simulink model "bicycle_model"  (R2021a)
settings: Solver=FixedStepDiscrete  StartTime=0.0  StopTime=365  FixedStep=0.05  RelTol=1e-3
values from neighbouring files (symbols this model uses):
  L = 2.2    [changing_ld.m]    (also in params.m)
  Ld = 10    [changing_ld.m]    (also in params.m = 5)
  v = 1.0    (= 1)    [changing_ld.m]    (also in params.m)
  waypoints = [       0    0 ... (first row only)    [changing_ld.m]    (also in params.m)
undefined symbols (not defined in the file or in its folder): DiscIntNeverNeededParam
settings Model: Creator=Sıla The Magnificent  LastModifiedBy=Sıla The Magnificent

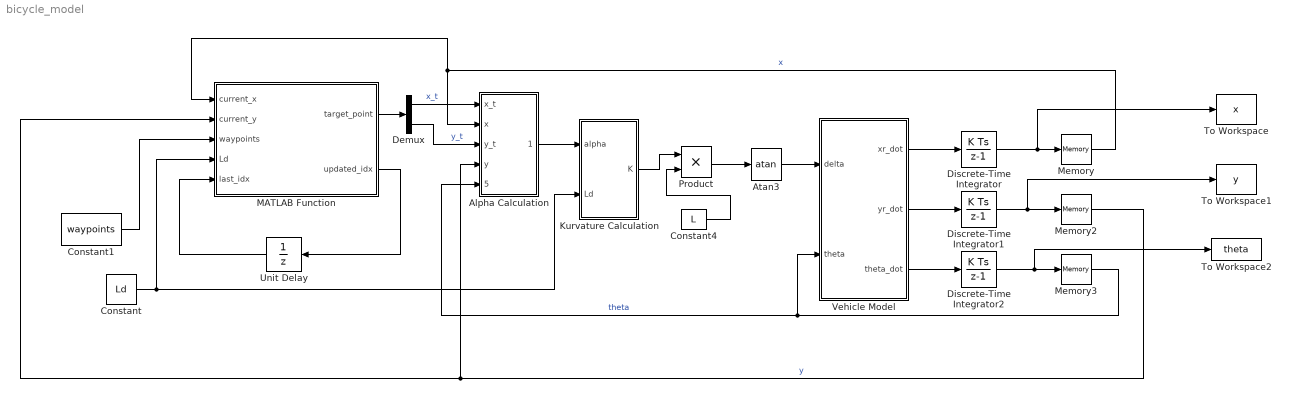
== system bicycle_model ==
  Alpha Calculation : Subsystem
  Atan3 : Trigonometry  Operator=atan
  Constant : Constant  Value=Ld
  Constant1 : Constant  Value=waypoints  SampleTime=0.05
  Constant4 : Constant  Value=L
  Demux : Demux  Outputs=2
  Discrete-Time Integrator : DiscreteIntegrator  SampleTime=0.05  ICPrevOutput=DiscIntNeverNeededParam  ICPrevScaledInput=DiscIntNeverNeededParam
  Discrete-Time Integrator1 : DiscreteIntegrator  SampleTime=0.05  ICPrevOutput=DiscIntNeverNeededParam  ICPrevScaledInput=DiscIntNeverNeededParam
  Discrete-Time Integrator2 : DiscreteIntegrator  SampleTime=0.05  ICPrevOutput=DiscIntNeverNeededParam  ICPrevScaledInput=DiscIntNeverNeededParam
  Kurvature Calculation : Subsystem
  MATLAB Function : MATLAB Function  TreatAsAtomicUnit=on  SystemSampleTime=0.05
  Memory : Memory  InheritSampleTime=on
  Memory2 : Memory  InheritSampleTime=on
  Memory3 : Memory  InheritSampleTime=on
  Product : Product
  To Workspace : ToWorkspace  VariableName=x  SaveFormat=Timeseries  SampleTime=-1
  To Workspace1 : ToWorkspace  VariableName=y  SaveFormat=Timeseries  SampleTime=-1
  To Workspace2 : ToWorkspace  VariableName=theta  SaveFormat=Timeseries  SampleTime=-1
  Unit Delay : UnitDelay  InitialCondition=2  SampleTime=0.05  HasFrameUpgradeWarning=on
  Vehicle Model : Subsystem
  wires:
  Vehicle Model/1(xr_dot) -> Discrete-Time Integrator/1
  Vehicle Model/2(yr_dot) -> Discrete-Time Integrator1/1
  Vehicle Model/3(theta_dot) -> Discrete-Time Integrator2/1
  Discrete-Time Integrator/1 -> To Workspace/1, Memory/1
  Memory/1 -> Alpha Calculation/2(x), MATLAB Function/1(current_x)  "x"
  Discrete-Time Integrator1/1 -> Memory2/1, To Workspace1/1
  Memory2/1 -> Alpha Calculation/4(y), MATLAB Function/2(current_y)  "y"
  Discrete-Time Integrator2/1 -> Memory3/1, To Workspace2/1
  Memory3/1 -> Vehicle Model/2(theta), Alpha Calculation/5(theta)  "theta"
  Product/1 -> Atan3/1
  Atan3/1 -> Vehicle Model/1(delta)
  Constant1/1 -> MATLAB Function/3(waypoints)
  Constant/1 -> MATLAB Function/4(Ld), Kurvature Calculation/2(Ld)
  MATLAB Function/2(updated_idx) -> Unit Delay/1
  Unit Delay/1 -> MATLAB Function/5(last_idx)
  MATLAB Function/1(target_point) -> Demux/1
  Demux/1 -> Alpha Calculation/1(x_t)  "x_t"
  Alpha Calculation/1(alpha) -> Kurvature Calculation/1(alpha)
  Demux/2 -> Alpha Calculation/3(y_t)  "y_t"
  Kurvature Calculation/1(K) -> Product/1
  Constant4/1 -> Product/2

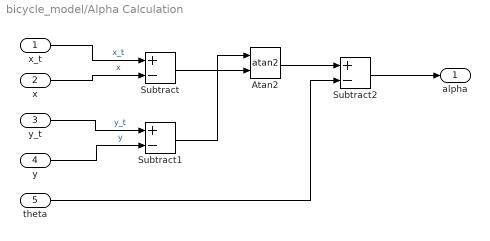
== system bicycle_model/Alpha Calculation ==
  x_t : Inport
  x : Inport  Port=2
  y_t : Inport  Port=3
  y : Inport  Port=4
  theta : Inport  Port=5
  Atan2 : Trigonometry  Operator=atan2
  Subtract : Sum  Inputs=+-
  Subtract1 : Sum  Inputs=+-
  Subtract2 : Sum  Inputs=+-
  alpha : Outport
  wires:
  x_t/1 -> Subtract/1  "x_t"
  Atan2/1 -> Subtract2/1
  x/1 -> Subtract/2  "x"
  y/1 -> Subtract1/2  "y"
  Subtract1/1 -> Atan2/1
  Subtract/1 -> Atan2/2
  Subtract2/1 -> alpha/1
  y_t/1 -> Subtract1/1  "y_t"
  theta/1 -> Subtract2/2

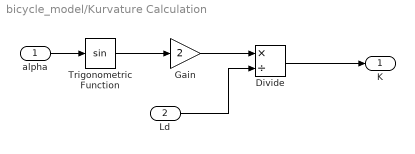
== system bicycle_model/Kurvature Calculation ==
  alpha : Inport
  Ld : Inport  Port=2
  Divide : Product  Inputs=*/
  Gain : Gain  Gain=2
  Trigonometric Function : Trigonometry
  K : Outport
  wires:
  Gain/1 -> Divide/1
  Ld/1 -> Divide/2
  Divide/1 -> K/1
  Trigonometric Function/1 -> Gain/1
  alpha/1 -> Trigonometric Function/1

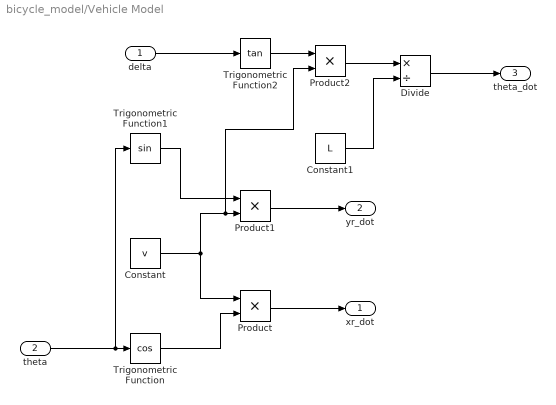
== system bicycle_model/Vehicle Model ==
  delta : Inport  OutMin=-0.5236  OutMax=0.5236
  theta : Inport  Port=2
  Constant : Constant  Value=v
  Constant1 : Constant  Value=L
  Divide : Product  Inputs=*/
  Product : Product
  Product1 : Product
  Product2 : Product
  Trigonometric Function : Trigonometry  Operator=cos
  Trigonometric Function1 : Trigonometry
  Trigonometric Function2 : Trigonometry  Operator=tan
  xr_dot : Outport
  yr_dot : Outport  Port=2
  theta_dot : Outport  Port=3
  wires:
  Trigonometric Function1/1 -> Product1/1
  Constant/1 -> Product2/2, Product1/2, Product/1
  Trigonometric Function/1 -> Product/2
  theta/1 -> Trigonometric Function1/1, Trigonometric Function/1
  delta/1 -> Trigonometric Function2/1
  Product/1 -> xr_dot/1
  Trigonometric Function2/1 -> Product2/1
  Product1/1 -> yr_dot/1
  Product2/1 -> Divide/1
  Constant1/1 -> Divide/2
  Divide/1 -> theta_dot/1

== matlab function bicycle_model/MATLAB Function ==
  data: current_x input; target_point output; current_y input; waypoints input; Ld input; updated_idx output; last_idx input
function [target_point, updated_idx] = getTargetPoint(current_x, current_y, waypoints, Ld, last_idx)
    
    target_point = waypoints(end, :);
    updated_idx = last_idx;

    for i = last_idx:size(waypoints, 1)
        dx = waypoints(i,1) - current_x;
        dy = waypoints(i,2) - current_y;
        distance = sqrt(dx^2 + dy^2);

        if distance >= Ld
            target_point = waypoints(i, :);
            updated_idx = i;
            break;
        end
    end
end
